simulink model "gm_uz_rs_flip_flop"  (R2021b)
settings: Solver=FixedStepDiscrete  StartTime=0.0  StopTime=10.0  RelTol=1e-3
libraries: simulink_extras x1
settings Model: Creator=valen  LastModifiedBy=valen
settings SolverCC: AlgebraicLoopSolver=TrustRegion
settings DataIOCC: LimitDataPoints=on  SaveOutput=off  SaveTime=off
settings OptimizationCC: BlockReduction=off  ConditionallyExecuteInputs=off  DefaultParameterBehavior=Inlined  LifeSpan=inf
settings DebuggingCC: AlgebraicLoopMsg=error  InheritedTsInSrcMsg=none  SingleTaskRateTransMsg=error  AllowSymbolicDim=off  StrictBusMsg=ErrorOnBusTreatedAsVector  SFUnexpectedBacktrackingDiag=warning  SFNoUnconditionalDefaultTransitionDiag=warning  SFExecutionAtInitializationDiag=none  SFMachineParentedDataDiag=warning  ArithmeticOperatorsInVariantConditions=warning
settings HardwareCC: ProdBitPerPointer=32  ProdBitPerSizeT=32  ProdBitPerPtrDiffT=32  ProdLargestAtomicFloat=None  ProdIntDivRoundTo=Undefined  ProdEndianess=Unspecified  ProdWordSize=32  ProdHWDeviceType=ASIC/FPGA->ASIC/FPGA  ProdEqTarget=off
settings SFSimCC: SimUseLocalCustomCode=off  CustomCodeUndefinedFunction=UseInterfaceOnly
settings RTWCC: RTWUseLocalCustomCode=off
settings CodeAppCC: StateflowObjectComments=on
settings GRTTargetCC: TargetLangStandard=C89/C90 (ANSI)
settings ConfigComp: CovScope=ReferencedModels  CovMetricSettings=dw  CovSaveCumulativeToWorkspaceVar=on  CovSaveSingleToWorkspaceVar=on  CovExternalEMLEnable=off  CovSFcnEnable=off

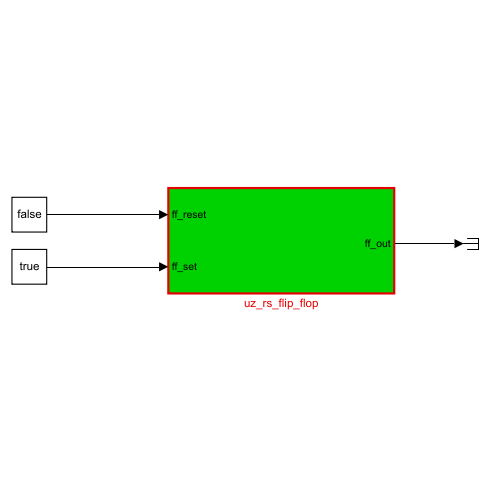
[thumbnail: Simulink's stored preview of the top-level diagram]
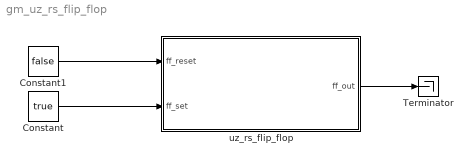
== system gm_uz_rs_flip_flop ==
  Constant : Constant  Value=true  SampleTime=1/1e8
  Constant1 : Constant  Value=false  SampleTime=1/1e8
  Terminator : Terminator
  uz_rs_flip_flop : Subsystem  TreatAsAtomicUnit=on
  wires:
  uz_rs_flip_flop/1(ff_out) -> Terminator/1
  Constant/1 -> uz_rs_flip_flop/2(ff_set)
  Constant1/1 -> uz_rs_flip_flop/1(ff_reset)

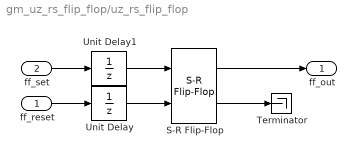
== system gm_uz_rs_flip_flop/uz_rs_flip_flop ==
  ff_reset : Inport
  ff_set : Inport  Port=2
  S-R Flip-Flop : simulink_extras/Flip Flops/S-R Flip-Flop  initial_condition=0
  Terminator : Terminator
  Unit Delay : UnitDelay  SampleTime=-1  HasFrameUpgradeWarning=on
  Unit Delay1 : UnitDelay  SampleTime=-1  HasFrameUpgradeWarning=on
  ff_out : Outport  VectorParamsAs1DForOutWhenUnconnected=off
  wires:
  S-R Flip-Flop/2 -> Terminator/1
  S-R Flip-Flop/1 -> ff_out/1
  Unit Delay1/1 -> S-R Flip-Flop/1
  Unit Delay/1 -> S-R Flip-Flop/2
  ff_reset/1 -> Unit Delay/1
  ff_set/1 -> Unit Delay1/1
